simulink model "ex2_2_4"  (R2023b)
settings: Solver=VariableStepAuto  StartTime=0.0  StopTime=10.0  RelTol=1e-3
libraries: dspsnks4 x1
settings Model: Creator=mariakahale  LastModifiedBy=mariakahale

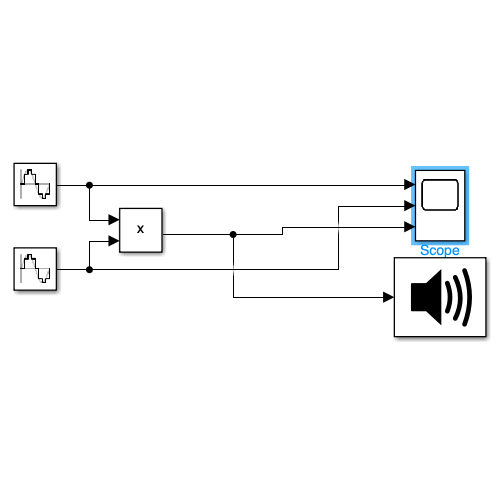
[thumbnail: Simulink's stored preview of the top-level diagram]
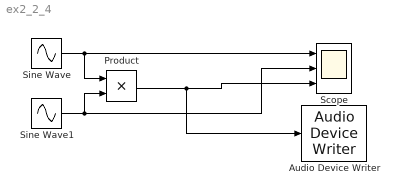
== system ex2_2_4 ==
  Audio Device Writer : dspsnks4/Audio Device Writer  Driver=CoreAudio  Device=Default  InheritSampleRate=on  SampleRate=44100  BitDepth=16-bit integer  BufferSize=4096  NumBuffers=10  DefaultOutputChannelMapping=on  OutputChannelMapping=1:2  OutputNumUnderrunSamples=off  DriverIdx=5  DeviceWarnFlag=''
  Product : Product
  Scope : Scope  NumInputPorts=3
  Sine Wave : Sin  Frequency=196350  SampleTime=1/48000
  Sine Wave1 : Sin  Frequency=3142  SampleTime=1/48000
  wires:
  Sine Wave/1 -> Product/1, Scope/1
  Sine Wave1/1 -> Scope/2, Product/2
  Product/1 -> Audio Device Writer/1, Scope/3
